simulink model "MINI_Simscape_Assignment_03"  (R2020b)
settings: Solver=FixedStepAuto  StartTime=0.0  StopTime=5  FixedStep=0.001  MaxStep=0.01  RelTol=1e-3
InitFcn:
  | parameters;
model workspace: external: MATLAB File /Users/toricolthurst/Documents/MATLAB/MINI_Simscape_Assingment_3/Simulation_DataFile.m (data not in the file)
values from neighbouring files (symbols this model uses):
  Butter_order = 4    [parameters.m]
  Butter_order_IMU = 8    [parameters.m]
undefined symbols (not defined in the file or in its folder): smiData, X, Y, Z
libraries: sm_lib x378, nesl_utility x72, dsparch4 x11, simulink x4
(part 8 of 8)

== matlab function MINI_Simscape_Assignment_03/MATLAB Function4 ==
  data: P_CoM_wholebody output; joint_angle input; P_CoM_part output
function [P_CoM_wholebody, P_CoM_part] = COM_FK(joint_angle)

% CoM Calculation code
% Input: joint Angles
% Output: 1) P_CoM_part: 3 x 17 matrix of CoM positions of each links. Each
%            column contains CoM position of each links with respect to the 
%            frame 0. [CoM_x; CoM_y; CoM_z;]
%
%         2) P_CoM_wholebody: 3x1 array of the position of the whole body
%            CoM [CoM_x; CoM_y; CoM_z;]

coder.extrinsic('-sync:on','DHparameter');
coder.extrinsic('-sync:on','TXYZ');
coder.extrinsic('-sync:on','RX');
coder.extrinsic('-sync:on','RY');
coder.extrinsic('-sync:on','RZ');

th1 = joint_angle(1); th3 = joint_angle(2); th5 = joint_angle(3);
th2 = joint_angle(4); th4 = joint_angle(5); th6 = joint_angle(6);
th7 = joint_angle(7); th9 = joint_angle(8); th11 = joint_angle(9); th13 = joint_angle(10); th15 = joint_angle(11);
th8 = joint_angle(12); th10 = joint_angle(13); th12 = joint_angle(14); th14 = joint_angle(15); th16 =joint_angle(16);

L_sh = 39; % Origin to arm roll joint
L_a1 = 18; % Shoulder bracket horizontal distance
L_a2 = 12; % Shoulder bracket vertical distance
L_a3 = 45; % Upper arm length
L_a4 = 72; % Lower arm length

L_by = 24; % Origin to pelvis vertical length
L_bz = 72; % Pelvis horizontal length
L_bx = 15; % Shoulder joint axis to Leg center (On Sagittal Plane)
L_l1 = 6;  % Pelvis Roll axis to pitch axis
L_l2 = 45; % Thigh Length
L_l3 = 42; % Shank Length
L_l4 = 31;  % Ankle Length


m_body = 250.48;
m_arm1 = 4.26;
m_arm2 = 23;
m_arm3 = 26.16;
m_leg1 = 19.9;
m_leg2 = 23;
m_leg3 = 8.99;
m_leg4 = 19.57;
m_leg5 = 36.53;

T_RH = zeros(4,4,4);
T_LH = zeros(4,4,4);
T_RF = zeros(4,4,6);
T_LF = zeros(4,4,6);

T_RH_all = zeros(4,4,4);
T_LH_all = zeros(4,4,4);
T_RF_all = zeros(4,4,6);
T_LF_all = zeros(4,4,6);

P_CoM_part_temp = zeros(4,17);
P_CoM_part = zeros(3,17)

% CoM Location
CoM_body = [-1.77; 0; -21.33];
CoM_RH_1 = [4.57; 0; -8.85];
CoM_RH_2 = [12.05; 0.97; -0.05];
CoM_RH_3 = [20; 1.29; 0.18];
CoM_LH_1 = [4.57; 0; -8.85];
CoM_LH_2 = [12.05; -0.97; -0.05];
CoM_LH_3 = [20; -1.29; 0.18];
CoM_RF_1 = [-1.22; -0.06; -1.47];
CoM_RF_2 = [32.95; -0.97; -0.05];
CoM_RF_3 = [17.90; -6.88; 0];
CoM_RF_4 = [-6.23; -1.76; 0.06];
CoM_RF_5 = [12.25; 8.01; 21.06];
CoM_LF_1 = [-1.22; 0.06; -1.47];
CoM_LF_2 = [32.95; 0.97; -0.05];
CoM_LF_3 = [17.90; 6.88; 0];
CoM_LF_4 = [-6.23; 1.76; 0.06];
CoM_LF_5 = [12.25; -8.01; 21.06];

% Right Hand
% DH parameter starts from arm origin at the shoulder
%    [a   alpha  d  theta]
DH_RH = [0, 0, 0, th1-(pi)/2;
    L_a2, (pi)/2, 0, (pi)/2+th3;
    L_a3, 0, 0, th5;
    L_a4, 0, 0, 0];

T_RH_all = DHparameter(DH_RH);
T_RH(:,:,1) = TXYZ(0,-(L_sh+L_a1),0)*RX((pi)/2)*T_RH_all(:,:,1);
T_RH(:,:,2) = T_RH(:,:,1)*T_RH_all(:,:,2);
T_RH(:,:,3) = T_RH(:,:,2)*T_RH_all(:,:,3);
T_RH(:,:,4) = T_RH(:,:,3)*T_RH_all(:,:,4);

P_CoM_part_temp(:,1) = T_RH(:,:,1)*[CoM_RH_1;1];
P_CoM_part_temp(:,2) = T_RH(:,:,2)*[CoM_RH_2;1];
P_CoM_part_temp(:,3) = T_RH(:,:,3)*[CoM_RH_3;1];

% Left Hand
% DH parameter starts from arm origin at the shoulder
% Modified DH
%    [a   alpha  d  theta]
DH_LH = [0, 0, 0, th2+(pi)/2;
    L_a2, -(pi)/2, 0, -(pi)/2+th4;
    L_a3, 0, 0, th6;
    L_a4, 0, 0, 0];

T_LH_all = DHparameter(DH_LH);
T_LH(:,:,1) = TXYZ(0,L_sh+L_a1,0)*RX(-(pi)/2)*T_LH_all(:,:,1);
T_LH(:,:,2) = T_LH(:,:,1)*T_LH_all(:,:,2);
T_LH(:,:,3) = T_LH(:,:,2)*T_LH_all(:,:,3);
T_LH(:,:,4) = T_LH(:,:,3)*T_LH_all(:,:,4);

P_CoM_part_temp(:,4) = T_LH(:,:,1)*[CoM_LH_1;1];
P_CoM_part_temp(:,5) = T_LH(:,:,2)*[CoM_LH_2;1];
P_CoM_part_temp(:,6) = T_LH(:,:,3)*[CoM_LH_3;1];


% Right Foot
% DH parameter starts from the hip roll joint
%    [a   alpha  d  theta]
DH_RF = [0, 0, 0, th7;
    L_l1,-(pi)/2, 0, th9;
    L_l2, 0, 0, th11;
    L_l3, pi, 0, th13;
    0, pi/2, 0, th15;
    L_l4, 0, 0, 0];

T_RF_all = DHparameter(DH_RF);
T_RF(:,:,1) = TXYZ(L_bx,-L_by,-L_bz)*RY((pi)/2)*T_RF_all(:,:,1);
T_RF(:,:,2) = T_RF(:,:,1)*T_RF_all(:,:,2);
T_RF(:,:,3) = T_RF(:,:,2)*T_RF_all(:,:,3);
T_RF(:,:,4) = T_RF(:,:,3)*T_RF_all(:,:,4);
T_RF(:,:,5) = T_RF(:,:,4)*T_RF_all(:,:,5);
T_RF(:,:,6) = T_RF(:,:,5)*T_RF_all(:,:,6);

P_CoM_part_temp(:,7) = T_RF(:,:,1)*[CoM_RF_1;1];
P_CoM_part_temp(:,8) = T_RF(:,:,2)*[CoM_RF_2;1];
P_CoM_part_temp(:,9) = T_RF(:,:,3)*[CoM_RF_3;1];
P_CoM_part_temp(:,10) = T_RF(:,:,4)*[CoM_RF_4;1];
P_CoM_part_temp(:,11) = T_RF(:,:,5)*[CoM_RF_5;1];

% Left Foot
% DH parameter starts from the hip roll joint
%    [a   alpha  d  theta]
DH_LF = [0, 0, 0, th8;
    L_l1,(pi)/2, 0, th10;
    L_l2, 0, 0, th12;
    L_l3, pi, 0, th14;
    0, -pi/2, 0, th16
    L_l4, 0, 0, 0];

T_LF_all = DHparameter(DH_LF);
T_LF(:,:,1) = TXYZ(L_bx,L_by,-L_bz)*RY((pi)/2)*T_LF_all(:,:,1);
T_LF(:,:,2) = T_LF(:,:,1)*T_LF_all(:,:,2);
T_LF(:,:,3) = T_LF(:,:,2)*T_LF_all(:,:,3);
T_LF(:,:,4) = T_LF(:,:,3)*T_LF_all(:,:,4);
T_LF(:,:,5) = T_LF(:,:,4)*T_LF_all(:,:,5);
T_LF(:,:,6) = T_LF(:,:,5)*T_LF_all(:,:,6);

P_CoM_part_temp(:,12) = T_LF(:,:,1)*[CoM_LF_1;1];
P_CoM_part_temp(:,13) = T_LF(:,:,2)*[CoM_LF_2;1];
P_CoM_part_temp(:,14) = T_LF(:,:,3)*[CoM_LF_3;1];
P_CoM_part_temp(:,15) = T_LF(:,:,4)*[CoM_LF_4;1];
P_CoM_part_temp(:,16) = T_LF(:,:,5)*[CoM_LF_5;1];
P_CoM_part_temp(:,17) = [CoM_body;1];
%% Calculate Wholebody COM

P_CoM_wholebody = (P_CoM_part_temp(1:3,17)*m_body ...
    + P_CoM_part_temp(1:3,1)*m_arm1 + P_CoM_part_temp(1:3,2)*m_arm2 + P_CoM_part_temp(1:3,3)*m_arm3 ...
    + P_CoM_part_temp(1:3,4)*m_arm1 + P_CoM_part_temp(1:3,5)*m_arm2 + P_CoM_part_temp(1:3,6)*m_arm3 ...
    + P_CoM_part_temp(1:3,7)*m_leg1 + P_CoM_part_temp(1:3,8)*m_leg2 + P_CoM_part_temp(1:3,9)*m_leg3 + P_CoM_part_temp(1:3,10)*m_leg4 + P_CoM_part_temp(1:3,11)*m_leg5 ...
    + P_CoM_part_temp(1:3,12)*m_leg1 + P_CoM_part_temp(1:3,13)*m_leg2 + P_CoM_part_temp(1:3,14)*m_leg3 + P_CoM_part_temp(1:3,15)*m_leg4 + P_CoM_part_temp(1:3,16)*m_leg5)...
    /(m_body + 2*(m_arm1 + m_arm2 + m_arm3)+ 2*(m_leg1 + m_leg2 + m_leg3 + m_leg4 + m_leg5));

P_CoM_part = P_CoM_part_temp(1:3,:);

== matlab function MINI_Simscape_Assignment_03/MATLAB Function5 ==
  data: p_x_both output; L_force input; p_y_both output; R_force input; L_x_pos input; L_y_pos input; R_x_pos input; R_y_pos input
function [p_x_both, p_y_both] = measured_ZMP_FK(L_force, R_force, L_x_pos, L_y_pos, R_x_pos, R_y_pos)

% ZMP Calculation code
% Input: L_force, R_force, L_x_pos, L_y_pos, R_x_pos, R_y_pos
% Output: p_x_both, p_y_both - ZMP position 

R_force_tot = sum(R_force);
L_force_tot = sum(L_force);
force_tot = R_force_tot + L_force_tot;

if R_force_tot == 0
    R_p_x = 0;
    R_p_y = 0;
else
    R_p_x = sum(R_x_pos.*R_force) / R_force_tot;
    R_p_y = sum(R_y_pos.*R_force) / R_force_tot;
end
    
if L_force_tot == 0
    L_p_x = 0;
    L_p_y = 0;
else
    L_p_x = sum(L_x_pos.*L_force) / L_force_tot;
    L_p_y = sum(L_y_pos.*L_force) / L_force_tot;
end

if force_tot == 0
    p_x_both = 0;
    p_y_both = 0;
else
    p_x_both = (R_p_x*R_force_tot + L_p_x*L_force_tot) / force_tot;
    p_y_both = (R_p_y*R_force_tot + L_p_y*L_force_tot) / force_tot;
end
